simulink model "part2_linear"  (Simulink 9.0)
settings: Solver=VariableStepAuto  StartTime=0.0  StopTime=70  RelTol=1e-3
values from neighbouring files (symbols this model uses):
  c = 0.25    [Lab2.m]    (also in lab2.m)
  g = 9.81    [Lab2.m]    (also in lab2.m)
  l = 2    [Lab2.m]    (also in lab2.m)
  m = 1    [Lab2.m]    (also in lab2.m)
settings Model: Creator=ee105-abq  LastModifiedBy=Charlene Shong
settings DataIOCC: SaveFormat=Dataset
settings OptimizationCC: LifeSpan=auto
settings DebuggingCC: UnderspecifiedInitializationDetection=Simplified  MergeDetectMultiDrivingBlocksExec=error  SFUnexpectedBacktrackingDiag=error  SFNoUnconditionalDefaultTransitionDiag=error  SFExecutionAtInitializationDiag=warning
settings HardwareCC: ProdBitPerPointer=64  ProdBitPerSizeT=64  ProdBitPerPtrDiffT=64  ProdLargestAtomicFloat=Float  ProdIntDivRoundTo=Zero  ProdEndianess=LittleEndian  ProdWordSize=64  ProdHWDeviceType=Intel->x86-64 (Windows64)
settings ModelReferenceCC: PropagateSignalLabelsOutOfModel=on
settings GRTTargetCC: TargetLangStandard=C99 (ISO)
settings ConfigComp: CovMetricSettings=dwe  CovHtmlReporting=off  CovSaveCumulativeToWorkspaceVar=off  CovSaveSingleToWorkspaceVar=off  CovExternalEMLEnable=on

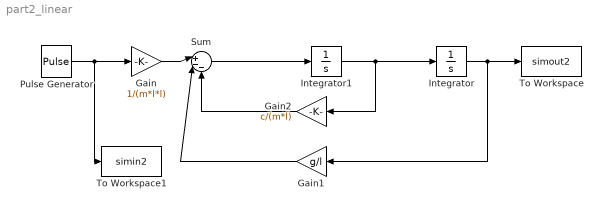
== system part2_linear ==
  Gain : Gain  Gain=1/(m*l*l)
  Gain1 : Gain  Gain=g/l
  Gain2 : Gain  Gain=c/(m*l)
  Integrator : Integrator
  Integrator1 : Integrator
  Pulse Generator : DiscretePulseGenerator  PulseType=Time based  Amplitude=10  Period=100  PulseWidth=0.2
  Sum : Sum  Inputs=|+--
  To Workspace : ToWorkspace  VariableName=simout2  SaveFormat=Timeseries  SampleTime=-1
  To Workspace1 : ToWorkspace  VariableName=simin2  SaveFormat=Timeseries  SampleTime=-1
  wires:
  Gain/1 -> Sum/1
  Integrator/1 -> Gain1/1, To Workspace/1
  Gain1/1 -> Sum/2
  Gain2/1 -> Sum/3
  Sum/1 -> Integrator1/1
  Integrator1/1 -> Gain2/1, Integrator/1
  Pulse Generator/1 -> To Workspace1/1, Gain/1
